simulink model "MultirotorModel"  (R2020b)
settings: Solver=VariableStepAuto  StartTime=0.0  StopTime=200  FixedStep=0.005  RelTol=1e-3  EnableMultiTasking=on
undefined symbols (not defined in the file): Controller, decyear, DiscIntNeverNeededParam, DroneMass, Dz, Earth, Gravity, initialConditions, Iz, leapyear, Nz, Pz, startFlightTime, UAVSampleTime, Vehicle, WGS84
libraries: pid_lib x10, uavalgslib x6, simulink x3, sharedutil x2, aerolibconvert2 x2, aerolibtransform2 x2, aerolibatmos2 x1, aerolibgravity2 x1, shared6dof x1, aerolibasang x1, mspsensorlib x1
(part 3 of 3)

== stateflow chart MultirotorModel/Guidance Logic/Full Guidance Logic/Guidance Stateflow/Guidance Mode Selector ==
  settings: updateMethod=DISCRETE  sampleTime=UAVSampleTime*4
  state GuidanceLogic
    state OnGround
    state Takeoff
    state WP
    state Orbit
    state Land
      state ToLand
      state Descend
      (default) -> ToLand
      ToLand -> Descend : [norm(Pose(1:2)-ToWP.position(1:2)) <= 2]
    (default) -> OnGround
    OnGround -> (junction 5) : [startFlight==1]
    Takeoff -> WP : [Pose(3) <= -ToWP.position(3)]
    GuidanceLogic -> (junction 5) : [hasChanged(mode)]
    (junction 5) -> Takeoff [order 1] : [mode == 1]
    (junction 5) -> (junction 12) [order 2]
    (junction 12) -> WP [order 1] : [mode==2]
    (junction 12) -> (junction 17) [order 2]
    (junction 17) -> Orbit [order 1] : [mode==3]
    (junction 17) -> (junction 22) [order 2]
    (junction 22) -> Land
    Land -> GuidanceLogic : [Pose(3)>=-0.1]{Status = 2}
  (default) -> GuidanceLogic
  data: sf_internal_action_state_placeholder_data local double size=1 =0; sf_internal_action_state_placeholder_data local double size=1 =0; sf_internal_action_state_placeholder_data local double size=1 =0; sf_internal_action_state_placeholder_data local double size=1 =0; sf_internal_action_state_placeholder_data local double size=1 =0; mode input; ToWP input Bus: uavPathManagerBus; InnerLoopCmds output Bus: innerLoopCmdsBus; Status output uint8; FromWP input Bus: uavPathManagerBus; Pose input; startFlight input
